simulink model "Battery_Electrothermal_Model_LT"  (R2025b)
settings: Solver=VariableStepAuto  StartTime=0.0  StopTime=t_end  MaxStep=0.1  RelTol=1e-3
InitFcn:
  | setup_battery_parameters
values from neighbouring files (symbols this model uses):
  Ambient_Temperature = 29.5    [setup_battery_parameters.m]
  Area = pi*21*70*10^(-6)+2*pi*(21/2)^2*10^(-6)    (= 0.00531086238089)    [setup_battery_parameters.m]
  C1C = flip([701	    701	    737	    768	    832	    782	    865	    890	    1031	1048	1048])    [setup_battery_parameters.m]
  C1D = flip([1087	1087	1038	887     1233	1215	1247	1366	1551	1211	1211])    [setup_battery_parameters.m]
  C2C = flip([1915	1915	1795	2005	1844	1682	1791	1995	1119	1880	1880])    [setup_battery_parameters.m]
  C2D = flip([2044	2044	2010	2634	2549	2450	2466	2716	1595	1396	1396])    [setup_battery_parameters.m]
  Capacity = 4    [setup_battery_parameters.m]
  ehc = [2.6e-04, 1.4e-04, 5.4e-05, -1.8e-05, -9.2e-05, -1.1e-04, -1.1e-04, -1.2e-04, -1.2e-04, -1.3e-04, -1.4e-04, -1.5e-04, -1.5e-04, -1.6e-04, -1.6e-04, -1.6e-04, -1.5e-04, -1.4e-04, -1.2e-04, -1.0e-04, -8.8e-05, -8.0e-05, -7.6e-05, -7.6e-05, -6.9e-05, -6.0e-05, -5.5e-05, -5.2e-05, -5.6e-05, -6.4e-05, -7.6e-05, -9.0e-05, -1.0e-04, -1.1e-04, -1.2e-04, -1.2e-04, -1.2e-04, -1.0e-04, -8.9e-05, -6.3e-05, -3 ...(+548 chars)    [setup_battery_parameters.m]
  Initial_SOC = 100    [setup_battery_parameters.m]
  OCV = flip([4.1	    4.05	3.96	3.87	3.79	3.72	3.63	3.53	3.46	3.29	3.07])    [setup_battery_parameters.m]
  R0C = flip([0.00748	0.00748	0.00743	0.00743	0.00748	0.00741	0.00744	0.00746	0.00746	0.00796	0.00796])    [setup_battery_parameters.m]
  R0D = flip([0.00750 0.00750 0.00739 0.00736 0.00738 0.00734 0.00730 0.00728 0.00737 0.00785 0.00785])    [setup_battery_parameters.m]
  R1C = flip([0.00170	0.00170	0.00150	0.00141	0.00137	0.00139	0.00136	0.00134	0.00118	0.00232	0.00232])    [setup_battery_parameters.m]
  R1D = flip([0.00168	0.00168	0.00159	0.00159	0.00175	0.00170	0.00160	0.00160	0.00178	0.00239	0.00239])    [setup_battery_parameters.m]
  R2C = flip([0.01233	0.01233	0.00794	0.00825	0.01080	0.01371	0.01193	0.00915	0.01579	0.01778	0.01778])    [setup_battery_parameters.m]
  R2D = flip([0.0083	0.0083	0.0098	0.0060	0.0077	0.0087	0.0087	0.0065	0.0193	0.0271	0.0271])    [setup_battery_parameters.m]
  SOC_vector = 0:10:100    [setup_battery_parameters.m]
  SOC_vector_100 = 0:1:100    [setup_battery_parameters.m]
libraries: fl_lib x14, nesl_utility x14, ee_lib x2
settings Model: Creator=truss  LastModifiedBy=truss

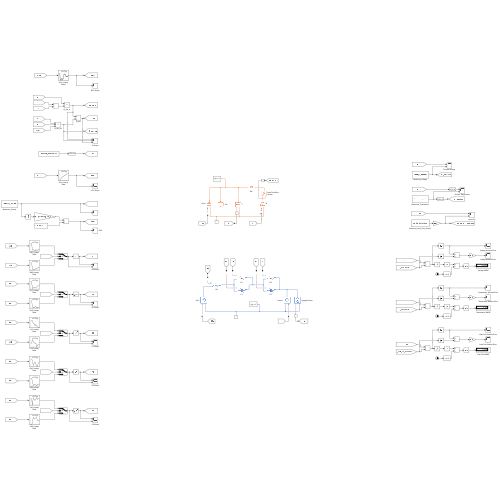
[thumbnail: Simulink's stored preview of the top-level diagram]
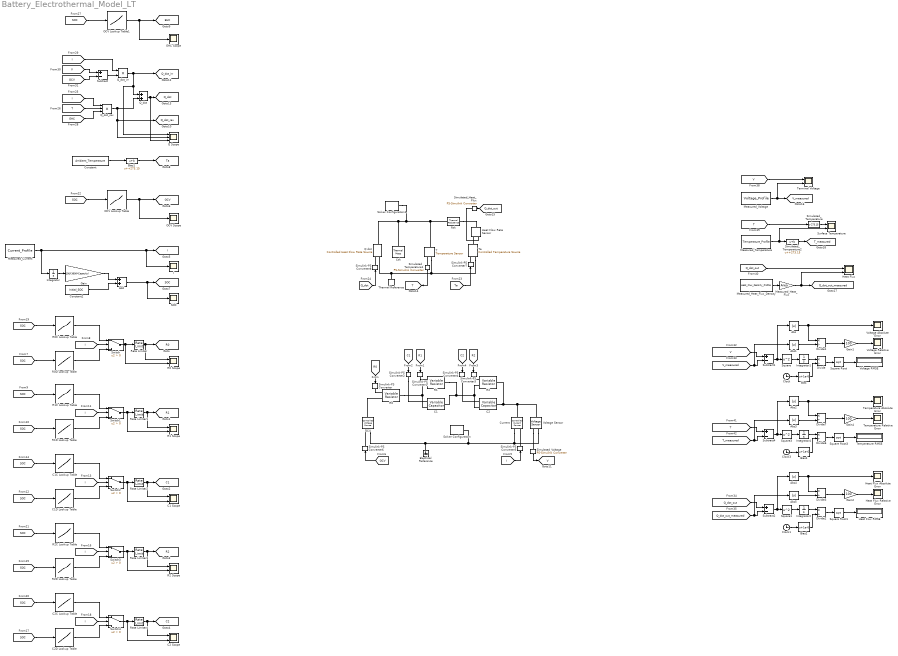
== system Battery_Electrothermal_Model_LT ==
  Abs{,1..5} (6 alike) : Abs  SaturateOnIntegerOverflow=off
  Add : Sum
  Bias : Bias  Bias=1e-6  SaturateOnIntegerOverflow=off
  Bias1 : Bias  Bias=+273.15  SaturateOnIntegerOverflow=off
  Bias2 : Bias  Bias=1e-6  SaturateOnIntegerOverflow=off
  Bias4 : Bias  Bias=1e-6  SaturateOnIntegerOverflow=off
  C1 : ee_lib/Passive/Variable Capacitor  prm=2  Cmin=1e-9 F  r=0 Ohm  v0=0 V  q0=0 C
      settings: InternalSimscapePortConfiguration="{\"Bottom\":[],\"Left\":[{\"id\":\"C\",\"label\":\"C\",\"type\":\"input\"},{\"id\":\"p\",\"label\":\"+\",\"type\":\"foundation.electrical.electrical\"}],\"Right\":[{\"id\":\"n\",\"label\":\"-\",\"type\":\"foundation.electrical.electrical\"}],\"Top\":[]}"
  C1 Scope : Scope  NumInputPorts=2
      settings: ActiveDisplayYMinimum=594.75184180346116  ActiveDisplayYMaximum=1657.23342376885  YLabel=C1 (F)  DataLoggingVariableName=ScopeData9
  C1C Lookup Table : Lookup_n-D  NumberOfTableDimensions=1  BreakpointsForDimension1=SOC_vector  BreakpointsForDimension2=[303.15]  Table=C1C  InternalRulePriority=Speed  RndMeth=Simplest
  C1D Lookup Table : Lookup_n-D  NumberOfTableDimensions=1  BreakpointsForDimension1=SOC_vector  BreakpointsForDimension2=[303.15]  Table=C1D  InternalRulePriority=Speed  RndMeth=Simplest
  C2 : ee_lib/Passive/Variable Capacitor  prm=2  Cmin=1e-9 F  r=0 Ohm  v0=0 V  q0=0 C
      settings: InternalSimscapePortConfiguration="{\"Bottom\":[],\"Left\":[{\"id\":\"C\",\"label\":\"C\",\"type\":\"input\"},{\"id\":\"p\",\"label\":\"+\",\"type\":\"foundation.electrical.electrical\"}],\"Right\":[{\"id\":\"n\",\"label\":\"-\",\"type\":\"foundation.electrical.electrical\"}],\"Top\":[]}"
  C2 Scope : Scope  NumInputPorts=2
      settings: ActiveDisplayYMinimum=973.96508512242644  ActiveDisplayYMaximum=2909.5251241384231  YLabel=C2 (F)  DataLoggingVariableName=ScopeData10
  C2C Lookup Table : Lookup_n-D  NumberOfTableDimensions=1  BreakpointsForDimension1=SOC_vector  BreakpointsForDimension2=[303.15]  Table=C2C  InternalRulePriority=Speed  RndMeth=Simplest
  C2D Lookup Table : Lookup_n-D  NumberOfTableDimensions=1  BreakpointsForDimension1=SOC_vector  BreakpointsForDimension2=[303.15]  Table=C2D  InternalRulePriority=Speed  RndMeth=Simplest
  Clock : Clock
  Clock1 : Clock
  Clock3 : Clock
  Constant : Constant  Value=Ambient_Temperature
  Constant2 : Constant  Value=Initial_SOC
  Cth : fl_lib/Thermal/Thermal Elements/Thermal Mass  mass_type=foundation.enum.constant_variable.constant  mass=Mass kg  sp_heat=Specific_Capacity_th J/(K*kg)  mass_min=1e-6 kg  num_ports=foundation.enum.numPorts2.one  m_specify=off  m_priority=High  m=1 kg  m_nominal_specify=off  m_nominal_value=1  m_nominal_unit=kg  T_specify=on  T_priority=High  T=Ambient_Temperature+273.15 K  T_nominal_specify=off  T_nominal_value=Ambient_Temperature  T_nominal_unit=K  Q_specify=off  Q_priority=None  Q=0 W  Q_nominal_specify=off  Q_nominal_value=1  Q_nominal_unit=W
  Current : fl_lib/Electrical/Electrical Sources/Controlled Current Source
  Divide{,1..3,6..7} (6 alike) : Product  Inputs=*/
  EHC Scope : Scope
      settings: ActiveDisplayYMinimum=-0.0024055623158018569  ActiveDisplayYMaximum=0.020050060842216715  YLabel=EHC (V/K)  DataLoggingVariableName=ScopeData13
  Electrical Reference : fl_lib/Electrical/Electrical Elements/Electrical Reference
  Gain : Gain  Gain=100/(3600*Capacity)
  Gain1 : Gain  Gain=100
  Gain2 : Gain  Gain=100
  Gain4 : Gain  Gain=100
  Heat Flow Rate Sensor : fl_lib/Thermal/Thermal Sensors/Heat Flow Rate Sensor
  Heat Flux : Scope  NumInputPorts=2
      settings: ActiveDisplayYMinimum=-0.06932137473654558  ActiveDisplayYMaximum=0.55269763983867093  YLabel=Heat Flux (W)  DataLoggingVariableName=ScopeData15
  Heat Flux Absolute Error : Scope
      settings: ActiveDisplayYMinimum=-0.051442008195510217  ActiveDisplayYMaximum=0.46297807375959432  YLabel=Voltage Error (V)  DataLoggingVariableName=ScopeData6
  Heat Flux RMSE : Display
  Heat Flux Relative Error : Scope
      settings: ActiveDisplayYMinimum=-3.4122486136681718  ActiveDisplayYMaximum=2.38369415726869  YLabel=Voltage Error (%)  DataLoggingVariableName=ScopeData18
  I : Scope
      settings: ActiveDisplayYMinimum=-27.990881  ActiveDisplayYMaximum=-7.9908810000000017  YLabel=Current (A)  DataLoggingVariableName=ScopeData7
  Integrator{,1..2,4} (4 alike) : Integrator
  Measured_Current : FromWorkspace  VariableName=Current_Profile  SampleTime=0.1
  Measured_Heat_Flux : Gain  Gain=Area
  Measured_Heat_Flux_Density : FromWorkspace  VariableName=Heat_Flux_Density_Profile  SampleTime=0.1
  Measured_Temperature : FromWorkspace  VariableName=Temperature_Profile  SampleTime=0.1
  Measured_Voltage : FromWorkspace  VariableName=Voltage_Profile  SampleTime=0.1
  OCV : fl_lib/Electrical/Electrical Sources/Controlled Voltage Source
  OCV Lookup Table : Lookup_n-D  NumberOfTableDimensions=1  BreakpointsForDimension1=SOC_vector  BreakpointsForDimension2=[303.15]  Table=OCV  InternalRulePriority=Speed  RndMeth=Simplest
  OCV Lookup Table1 : Lookup_n-D  NumberOfTableDimensions=1  BreakpointsForDimension1=SOC_vector_100  BreakpointsForDimension2=[303.15]  Table=ehc  InternalRulePriority=Speed  RndMeth=Simplest
  OCV Scope : Scope
      settings: ActiveDisplayYMinimum=-0.68269814488587888  ActiveDisplayYMaximum=4.6314109049873196  YLabel=OCV (V)  DataLoggingVariableName=ScopeData12
  Q Scope : Scope  NumInputPorts=3
      settings: ActiveDisplayYMinimum=-9.0795668867922767  ActiveDisplayYMaximum=11.422147436319515  YLabel=Heat Generation (W)  DataLoggingVariableName=ScopeData14
  Q dot : fl_lib/Thermal/Thermal Sources/Controlled Heat Flow Rate Source
  Q_dot : Sum
  Q_dot_irr : Product
  Q_dot_rev : Product  Inputs=3
  R0 : fl_lib/Electrical/Electrical Elements/Variable Resistor  Rmin=0 Ohm  thermalEnable=false  thermal_mass=1 J/K  i_specify=off  i_priority=None  i=0 A  i_nominal_specify=off  i_nominal_value=1  i_nominal_unit=A  v_specify=off  v_priority=None  v=0 V  v_nominal_specify=off  v_nominal_value=1  v_nominal_unit=V  T_specify=off  T_priority=None  T=300 K  T_nominal_specify=off  T_nominal_value=1  T_nominal_unit=K
  R0 Scope : Scope  NumInputPorts=2
      settings: ActiveDisplayYMinimum=0.0065  ActiveDisplayYMaximum=0.0085  YLabel=R0 (Ohm)  DataLoggingVariableName=ScopeData2
  R0C Lookup Table : Lookup_n-D  NumberOfTableDimensions=1  BreakpointsForDimension1=SOC_vector  BreakpointsForDimension2=[303.15]  Table=R0C  InternalRulePriority=Speed  RndMeth=Simplest
  R0D Lookup Table : Lookup_n-D  NumberOfTableDimensions=1  BreakpointsForDimension1=SOC_vector  BreakpointsForDimension2=[303.15]  Table=R0D  InternalRulePriority=Speed  RndMeth=Simplest
  R1 : fl_lib/Electrical/Electrical Elements/Variable Resistor  Rmin=0 Ohm  thermalEnable=false  thermal_mass=1 J/K  i_specify=off  i_priority=None  i=0 A  i_nominal_specify=off  i_nominal_value=1  i_nominal_unit=A  v_specify=off  v_priority=None  v=0 V  v_nominal_specify=off  v_nominal_value=1  v_nominal_unit=V  T_specify=off  T_priority=None  T=300 K  T_nominal_specify=off  T_nominal_value=1  T_nominal_unit=K
  R1 Scope : Scope  NumInputPorts=2
      settings: ActiveDisplayYMinimum=0.0010287599658838876  ActiveDisplayYMaximum=0.0025412488926795681  YLabel=R1 (Ohm)  DataLoggingVariableName=ScopeData8
  R1C Lookup Table : Lookup_n-D  NumberOfTableDimensions=1  BreakpointsForDimension1=SOC_vector  BreakpointsForDimension2=[303.15]  Table=R1C  InternalRulePriority=Speed  RndMeth=Simplest
  R1D Lookup Table : Lookup_n-D  NumberOfTableDimensions=1  BreakpointsForDimension1=SOC_vector  BreakpointsForDimension2=[303.15]  Table=R1D  InternalRulePriority=Speed  RndMeth=Simplest
  R2 : fl_lib/Electrical/Electrical Elements/Variable Resistor  Rmin=0 Ohm  thermalEnable=false  thermal_mass=1 J/K  i_specify=off  i_priority=None  i=0 A  i_nominal_specify=off  i_nominal_value=1  i_nominal_unit=A  v_specify=off  v_priority=None  v=0 V  v_nominal_specify=off  v_nominal_value=1  v_nominal_unit=V  T_specify=off  T_priority=None  T=300 K  T_nominal_specify=off  T_nominal_value=1  T_nominal_unit=K
  R2 Scope : Scope  NumInputPorts=2
      settings: ActiveDisplayYMinimum=0.0033625496855732391  ActiveDisplayYMaximum=0.029737494479380754  YLabel=R2 (Ohm)  DataLoggingVariableName=ScopeData11
  R2C Lookup Table : Lookup_n-D  NumberOfTableDimensions=1  BreakpointsForDimension1=SOC_vector  BreakpointsForDimension2=[303.15]  Table=R2C  InternalRulePriority=Speed  RndMeth=Simplest
  R2D Lookup Table : Lookup_n-D  NumberOfTableDimensions=1  BreakpointsForDimension1=SOC_vector  BreakpointsForDimension2=[303.15]  Table=R2D  InternalRulePriority=Speed  RndMeth=Simplest
  Rate Limiter{,1..4} (5 alike) : RateLimiter  RisingSlewLimit=1000  FallingSlewLimit=-1000  SampleTimeMode=inherited
  Rth : fl_lib/Thermal/Thermal Elements/Thermal Resistance  resistance=Ambient_Resistance_th K/W  T_specify=off  T_priority=None  T=0 K  T_nominal_specify=off  T_nominal_value=1  T_nominal_unit=K  Q_specify=off  Q_priority=None  Q=0 W  Q_nominal_specify=off  Q_nominal_value=1  Q_nominal_unit=W
  SOC : Scope
      settings: ActiveDisplayYMinimum=-176.66897590471157  ActiveDisplayYMaximum=130.74099732274573  YLabel=SOC (%)
  Simulated_Heat_Flux : nesl_utility/PS-Simulink Converter  PhysicalDomain=network_engine_domain  SubClassName=ps_output  LeftPortType=input  RightPortType=output  PseudoPeriodic=off  Frequencies=[]  VectorFormat=inherit  Unit=inherit  AffineConversion=off
  Simulated_Temperature : Bias  Bias=-273.15  SaturateOnIntegerOverflow=off
  Simulated_Temperature1 : nesl_utility/PS-Simulink Converter  PhysicalDomain=network_engine_domain  SubClassName=ps_output  LeftPortType=input  RightPortType=output  PseudoPeriodic=off  Frequencies=[]  VectorFormat=inherit  Unit=inherit  AffineConversion=off
  Simulated_Temperature2 : Bias  Bias=+273.15  SaturateOnIntegerOverflow=off
  Simulated_Voltage : nesl_utility/PS-Simulink Converter  PhysicalDomain=network_engine_domain  SubClassName=ps_output  LeftPortType=input  RightPortType=output  PseudoPeriodic=off  Frequencies=[]  VectorFormat=inherit  Unit=inherit  AffineConversion=off
  Simulink-PS Converter{,1..4,8} (6 alike) : nesl_utility/Simulink-PS Converter  PhysicalDomain=network_engine_domain  SubClassName=ps_input  LeftPortType=input  RightPortType=output  PseudoPeriodic=off  Frequencies=[]  NoiseDistribution=none  NoiseParameters=[]  Unit=1  AffineConversion=off  FilteringAndDerivatives=provide  SimscapeFilterOrder=1  InputFilterTimeConstant=0.001  UdotUserProvided=0
  Simulink-PS Converter5 : nesl_utility/Simulink-PS Converter  PhysicalDomain=network_engine_domain  SubClassName=ps_input  LeftPortType=input  RightPortType=output  PseudoPeriodic=off  Frequencies=[]  NoiseDistribution=none  NoiseParameters=[]  Unit=A  AffineConversion=off  FilteringAndDerivatives=filter  SimscapeFilterOrder=1  InputFilterTimeConstant=0.001  UdotUserProvided=0
  Simulink-PS Converter6 : nesl_utility/Simulink-PS Converter  PhysicalDomain=network_engine_domain  SubClassName=ps_input  LeftPortType=input  RightPortType=output  PseudoPeriodic=off  Frequencies=[]  NoiseDistribution=none  NoiseParameters=[]  Unit=V  AffineConversion=off  FilteringAndDerivatives=provide  SimscapeFilterOrder=1  InputFilterTimeConstant=0.001  UdotUserProvided=0
  Simulink-PS Converter7 : nesl_utility/Simulink-PS Converter  PhysicalDomain=network_engine_domain  SubClassName=ps_input  LeftPortType=input  RightPortType=output  PseudoPeriodic=off  Frequencies=[]  NoiseDistribution=none  NoiseParameters=[]  Unit=K  AffineConversion=off  FilteringAndDerivatives=provide  SimscapeFilterOrder=1  InputFilterTimeConstant=0.001  UdotUserProvided=0
  Solver Configuration : nesl_utility/Solver Configuration  PhysicalDomain=network_engine_domain  SubClassName=solver  LeftPortType=input  RightPortType=generic  Tones=[]  Harmonics=[]  SimulateNoise=off  Profile=off  UseLocalSampling=off  EnableSwitchedLinearOptims=on  FrequencyDomain=off  UseCCode=off  RelTol=0.001  AbsTol=0.001  MinStep=1e-09  ToWorkspace=off  RevertToSquareIcSolve=off  NumHomotopyIterations=100  PhasorMode=off  PhasorModeNumHarmonics=1  ConsistencySolver=NEWTON_XTOL_AFTER_FTOL  IndexReductionMethod=DerivativeReplacement  DoDC=off  ResidualTolerance=1e-09  ConsistencyTolSource=GLOBAL  ConsistencyAbsTol=0.001  ConsistencyRelTol=0.001  ConsistencyTolFactor=0.001  UseLocalSolver=off  LocalSolverChoice=NE_BACKWARD_EULER_ADVANCER  ResolveIndetEquations=on  FunctionEvalNumThread=1  LocalSolverSampleTime=0.001  DoFixedCost=off  MaxNonlinIter=3  MaxModeIter=2  ComputeImpulses=off  ImpulseIterations=2  LinearAlgebra=auto  LinearAlgebraNumThread=0  EquationFormulation=NE_TIME_EF  DelaysMemoryBudget=1024  AutomaticFiltering=on  FilteringTimeConstant=0.001  PartitionStorageMethod=AS_NEEDED  PartitionMemoryBudget=1024  PartitionMethod=ROBUST  MultibodyUseLocalSolver=off  MultibodyLocalSolverChoice=ODE1  MultibodyLocalSolverSampleTime=0.001
  Solver Configuration1 : nesl_utility/Solver Configuration  PhysicalDomain=network_engine_domain  SubClassName=solver  LeftPortType=input  RightPortType=generic  Tones=[]  Harmonics=[]  SimulateNoise=off  Profile=off  UseLocalSampling=off  EnableSwitchedLinearOptims=on  FrequencyDomain=off  UseCCode=off  RelTol=0.001  AbsTol=0.001  MinStep=1e-09  ToWorkspace=off  RevertToSquareIcSolve=off  NumHomotopyIterations=100  PhasorMode=off  PhasorModeNumHarmonics=1  ConsistencySolver=NEWTON_XTOL_AFTER_FTOL  IndexReductionMethod=DerivativeReplacement  DoDC=off  ResidualTolerance=1e-09  ConsistencyTolSource=GLOBAL  ConsistencyAbsTol=0.001  ConsistencyRelTol=0.001  ConsistencyTolFactor=0.001  UseLocalSolver=off  LocalSolverChoice=NE_BACKWARD_EULER_ADVANCER  ResolveIndetEquations=on  FunctionEvalNumThread=1  LocalSolverSampleTime=0.001  DoFixedCost=off  MaxNonlinIter=3  MaxModeIter=2  ComputeImpulses=off  ImpulseIterations=2  LinearAlgebra=auto  LinearAlgebraNumThread=0  EquationFormulation=NE_TIME_EF  DelaysMemoryBudget=1024  AutomaticFiltering=on  FilteringTimeConstant=0.001  PartitionStorageMethod=AS_NEEDED  PartitionMemoryBudget=1024  PartitionMethod=ROBUST  MultibodyUseLocalSolver=off  MultibodyLocalSolverChoice=ODE1  MultibodyLocalSolverSampleTime=0.001
  Square : Math  Operator=square
  Square Root : Sqrt
  Square Root1 : Sqrt
  Square Root3 : Sqrt
  Square1 : Math  Operator=square
  Square3 : Math  Operator=square
  Subtract{,1..2,4} (4 alike) : Sum  Inputs=+-
  Surface Temperature : Scope  NumInputPorts=2
      settings: ActiveDisplayYMinimum=27.837639063293516  ActiveDisplayYMaximum=43.62809695635935  YLabel=Temperature (C)  DataLoggingVariableName=ScopeData4
  Switch{,1..4} (5 alike) : Switch  Criteria=u2 > Threshold  SaturateOnIntegerOverflow=off  InputSameDT=off
  T : fl_lib/Thermal/Thermal Sensors/Temperature Sensor  temperature_measure=foundation.enum.MeasurementReference.difference
  Ta : fl_lib/Thermal/Thermal Sources/Controlled Temperature Source
  Temperature Absolute Error : Scope
      settings: ActiveDisplayYMinimum=-0.58059208736482038  ActiveDisplayYMaximum=5.4573305105264893  YLabel=Voltage Error (V)  DataLoggingVariableName=ScopeData3
  Temperature RMSE : Display
  Temperature Relative Error : Scope
      settings: ActiveDisplayYMinimum=-3.4122486136681718  ActiveDisplayYMaximum=2.38369415726869  YLabel=Voltage Error (%)  DataLoggingVariableName=ScopeData5
  Terminal Voltage : Scope  NumInputPorts=2
      settings: ActiveDisplayYMinimum=2.6829079055525336  ActiveDisplayYMaximum=4.3146585594547195  YLabel=Voltage (V)
  Thermal Reference : fl_lib/Thermal/Thermal Elements/Thermal Reference
  Voltage Absolute Error : Scope
      settings: ActiveDisplayYMinimum=-0.044649582222888611  ActiveDisplayYMaximum=0.40184624000599756  YLabel=Voltage Error (V)  DataLoggingVariableName=ScopeData16
  Voltage RMSE : Display
  Voltage Relative Error : Scope
      settings: ActiveDisplayYMinimum=-1.3629298602835351  ActiveDisplayYMaximum=12.266368742551819  YLabel=Voltage Error (%)  DataLoggingVariableName=ScopeData17
  Voltage Sensor : fl_lib/Electrical/Electrical Sensors/Voltage Sensor
  tag scope: C1=global, C2=global, EHC=global, I=global, OCV=global, Q_dot=global, Q_dot_irr=global, Q_dot_out=global, Q_dot_out_measured=global, Q_dot_rev=global, R0=global, R1=global, R2=global, SOC=global, T=global, T_measured=global, Ta=global, V=global, V_measured=global
  wires:
  [R0] -> Simulink-PS Converter/1
  [R1] -> Simulink-PS Converter1/1
  [C1] -> Simulink-PS Converter2/1
  [C2] -> Simulink-PS Converter4/1
  [R2] -> Simulink-PS Converter3/1
  Simulated_Voltage/1 -> [V]
  [I] -> Simulink-PS Converter5/1
  [OCV] -> Simulink-PS Converter6/1
  Integrator/1 -> Gain/1
  Gain/1 -> Add/1
  Constant2/1 -> Add/2
  Add/1 -> SOC/1, [SOC]
  [SOC] -> R0D Lookup Table/1
  [SOC] -> R0C Lookup Table/1
  [SOC] -> OCV Lookup Table/1
  OCV Lookup Table/1 -> OCV Scope/1, [OCV]
  Measured_Current/1 -> Integrator/1, I/1, [I]
  R0C Lookup Table/1 -> Switch/1
  R0D Lookup Table/1 -> Switch/3
  [I] -> Switch/2
  Switch/1 -> R0 Scope/2, Rate Limiter/1
  Rate Limiter/1 -> R0 Scope/1, [R0]
  Switch1/1 -> R1 Scope/2, Rate Limiter1/1
  R1D Lookup Table/1 -> Switch1/3
  Rate Limiter1/1 -> R1 Scope/1, [R1]
  [I] -> Switch1/2
  R1C Lookup Table/1 -> Switch1/1
  [SOC] -> R1D Lookup Table/1
  [SOC] -> R1C Lookup Table/1
  Rate Limiter2/1 -> C1 Scope/1, [C1]
  [SOC] -> C1C Lookup Table/1
  C1C Lookup Table/1 -> Switch2/1
  [I] -> Switch2/2
  [SOC] -> C1D Lookup Table/1
  C1D Lookup Table/1 -> Switch2/3
  Switch2/1 -> C1 Scope/2, Rate Limiter2/1
  Rate Limiter4/1 -> C2 Scope/1, [C2]
  Switch4/1 -> C2 Scope/2, Rate Limiter4/1
  C2C Lookup Table/1 -> Switch4/1
  C2D Lookup Table/1 -> Switch4/3
  [I] -> Switch4/2
  [SOC] -> C2D Lookup Table/1
  [SOC] -> C2C Lookup Table/1
  Rate Limiter3/1 -> R2 Scope/1, [R2]
  [SOC] -> R2C Lookup Table/1
  R2C Lookup Table/1 -> Switch3/1
  [I] -> Switch3/2
  [SOC] -> R2D Lookup Table/1
  R2D Lookup Table/1 -> Switch3/3
  Switch3/1 -> R2 Scope/2, Rate Limiter3/1
  [Ta] -> Simulink-PS Converter7/1
  [Q_dot] -> Simulink-PS Converter8/1
  Constant/1 -> Bias1/1
  Simulated_Temperature1/1 -> [T]
  Bias1/1 -> [Ta]
  [SOC] -> OCV Lookup Table1/1
  OCV Lookup Table1/1 -> EHC Scope/1, [EHC]
  [I] -> Q_dot_rev/1
  [EHC] -> Q_dot_rev/3
  [T] -> Q_dot_rev/2
  Q_dot_rev/1 -> Q Scope/2, [Q_dot_rev], Q_dot/2
  [V] -> Subtract/1
  [OCV] -> Subtract/2
  [I] -> Q_dot_irr/1
  Subtract/1 -> Q_dot_irr/2
  Q_dot_irr/1 -> [Q_dot_irr], Q Scope/1, Q_dot/1
  Q_dot/1 -> Q Scope/3, [Q_dot]
  Simulated_Heat_Flux/1 -> [Q_dot_out]
  [V] -> Subtract1/1
  [V_measured] -> Abs1/1, Subtract1/2
  Subtract1/1 -> Abs/1, Square/1
  Square/1 -> Integrator1/1
  Integrator1/1 -> Divide/1
  Clock/1 -> Bias/1
  Bias/1 -> Divide/2
  Divide/1 -> Square Root/1
  Square Root/1 -> Voltage RMSE/1
  Divide1/1 -> Gain1/1
  Gain1/1 -> Voltage Relative Error/1
  [V] -> Terminal Voltage/1
  Measured_Voltage/1 -> [V_measured], Terminal Voltage/2
  Simulated_Temperature/1 -> Surface Temperature/1
  Simulated_Temperature2/1 -> [T_measured]
  Measured_Temperature/1 -> Surface Temperature/2, Simulated_Temperature2/1
  [T] -> Simulated_Temperature/1
  Measured_Heat_Flux/1 -> Heat Flux/2, [Q_dot_out_measured]
  Measured_Heat_Flux_Density/1 -> Measured_Heat_Flux/1
  [Q_dot_out] -> Heat Flux/1
  Abs/1 -> Divide1/1, Voltage Absolute Error/1
  Abs1/1 -> Divide1/2
  Abs2/1 -> Divide7/1, Temperature Absolute Error/1
  Abs3/1 -> Divide7/2
  [T] -> Subtract4/1
  [T_measured] -> Abs3/1, Subtract4/2
  Subtract4/1 -> Abs2/1, Square3/1
  Divide6/1 -> Square Root3/1
  Divide7/1 -> Gain4/1
  Clock3/1 -> Bias4/1
  Gain4/1 -> Temperature Relative Error/1
  Integrator4/1 -> Divide6/1
  Square Root3/1 -> Temperature RMSE/1
  Bias4/1 -> Divide6/2
  Square3/1 -> Integrator4/1
  Gain2/1 -> Heat Flux Relative Error/1
  Square Root1/1 -> Heat Flux RMSE/1
  Integrator2/1 -> Divide2/1
  Square1/1 -> Integrator2/1
  Bias2/1 -> Divide2/2
  Subtract2/1 -> Abs4/1, Square1/1
  Divide3/1 -> Gain2/1
  [Q_dot_out] -> Subtract2/1
  [Q_dot_out_measured] -> Abs5/1, Subtract2/2
  Abs4/1 -> Divide3/1, Heat Flux Absolute Error/1
  Abs5/1 -> Divide3/2
  Clock1/1 -> Bias2/1
  Divide2/1 -> Square Root1/1
  connections:
  OCV/LConn1 -- R0/LConn2
  R2/LConn2 -- C2/LConn2 -- C1/RConn1 -- R1/RConn1
  Voltage Sensor/LConn1 -- Current/LConn1 -- C2/RConn1 -- R2/RConn1
  OCV/RConn2 -- Current/RConn2 -- Voltage Sensor/RConn2 -- Solver Configuration/RConn1 -- Electrical Reference/LConn1
  Simulink-PS Converter/RConn1 -- R0/LConn1
  Simulink-PS Converter1/RConn1 -- R1/LConn1
  Simulink-PS Converter2/RConn1 -- C1/LConn1
  C2/LConn1 -- Simulink-PS Converter4/RConn1
  R2/LConn1 -- Simulink-PS Converter3/RConn1
  Simulink-PS Converter6/RConn1 -- OCV/RConn1
  Simulink-PS Converter5/RConn1 -- Current/RConn1
  Voltage Sensor/RConn1 -- Simulated_Voltage/LConn1
  R0/RConn1 -- C1/LConn2 -- R1/LConn2
  Q dot/LConn1 -- T/LConn1 -- Rth/LConn1 -- Solver Configuration1/RConn1 -- Cth/LConn1
  Thermal Reference/LConn1 -- Ta/RConn2 -- T/RConn1 -- Q dot/RConn2
  Rth/RConn1 -- Heat Flow Rate Sensor/LConn1
  Simulink-PS Converter7/RConn1 -- Ta/RConn1
  Simulink-PS Converter8/RConn1 -- Q dot/RConn1
  Simulated_Temperature1/LConn1 -- T/RConn2
  Heat Flow Rate Sensor/RConn2 -- Ta/LConn1
  Heat Flow Rate Sensor/RConn1 -- Simulated_Heat_Flux/LConn1
